simulink model "Test"  (R2017b)
settings: Solver=VariableStepAuto  StartTime=0.0  StopTime=6000  RelTol=1e-3
values from neighbouring files (symbols this model uses):
  C = tf([Kp Ki],[1 0])    [RunMe_SMPC.m]
  sys_ex = sys([iOMEGA0 iROOTMOOP], iTHETA0)    [RunMe_SMPC.m]
settings Model: Creator=sebastiaanmuld  LastModifiedBy=sebastiaanmuld

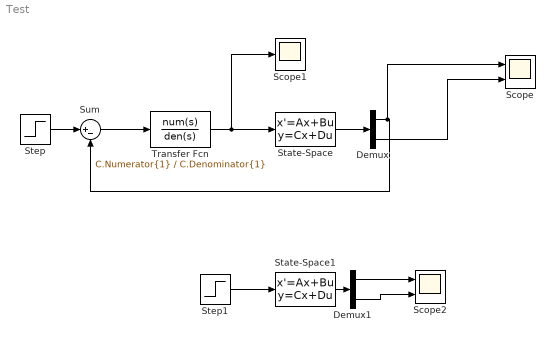
== system Test ==
  Demux : Demux  Outputs=2
  Demux1 : Demux  Outputs=2
  Scope : Scope  NumInputPorts=2
  Scope1 : Scope
  Scope2 : Scope  NumInputPorts=2
  State-Space : StateSpace  A=sys_ex.A  B=sys_ex.B  C=sys_ex.C  D=sys_ex.D  InitialCondition=0
  State-Space1 : StateSpace  A=sys_ex.A  B=sys_ex.B  C=sys_ex.C  D=sys_ex.D  InitialCondition=0
  Step : Step  After=0.1  SampleTime=0
  Step1 : Step  After=0.1  SampleTime=0
  Sum : Sum  Inputs=|+-
  Transfer Fcn : TransferFcn  Numerator=C.Numerator{1}  Denominator=C.Denominator{1}
  wires:
  Transfer Fcn/1 -> Scope1/1, State-Space/1
  Step/1 -> Sum/1
  Sum/1 -> Transfer Fcn/1
  State-Space/1 -> Demux/1
  Demux/1 -> Scope/1, Sum/2
  Demux/2 -> Scope/2
  Step1/1 -> State-Space1/1
  State-Space1/1 -> Demux1/1
  Demux1/1 -> Scope2/1
  Demux1/2 -> Scope2/2
